simulink model "Final_project"  (R2015b)
settings: Solver=FixedStepDiscrete  StartTime=0.0  StopTime=10.0  RelTol=1e-3
InitFcn:
  | parameters
values from neighbouring files (symbols this model uses):
  Ak = 100    [parameters.m]
  b = 100    [parameters.m]
  dT = 0.01    [parameters.m]
  H = 20    [parameters.m]
  m = 2000    [parameters.m]
  pot_gain = .33    (= 0.33)    [parameters.m]
  pot_offset = 512    [parameters.m]
  R = 1/5    (= 0.2)    [parameters.m]
  V_Ki = 50    [parameters.m]
  V_Kp = 5000    [parameters.m]
undefined symbols (not defined in the file or in its folder): A10, A13, A14, AN0, AN12, B, B13, B4, B6, C6, D, D11, D4, DiscIntNeverNeededParam, F17, F3, F4, G4, H4, L3, PA10, PA11, PA12, PA13, PA14, PA5, PA6, PA7, PA8, PA9, PB10, PB7, PC6, PD10, PD11, PG4, R10, R16, R5, R8, T15
libraries: Conv_Lib x54, rappid_564xl_ec_toolbox x34, Veh_Sim x9, simulink x4, U_of_M_5643_blockset x1
(part 2 of 2)

== system Final_project/High Level Design/Automatic Cruise Control/Speed Ctrl/PI/My Discrete Integrator ==
  X_dot : Inport
  Gain : Gain  Gain=dT  SaturateOnIntegerOverflow=on  OutDataTypeStr=Inherit: Same as input  ParamDataTypeStr=Inherit: Same as input
  Sum : Sum  Inputs=|++  SaturateOnIntegerOverflow=on  InputSameDT=on  OutDataTypeStr=Inherit: Same as first input
  Unit Delay : UnitDelay  SampleTime=-1
  X : Outport
  wires:
  Unit Delay/1 -> X/1, Sum/2
  Sum/1 -> Unit Delay/1
  X_dot/1 -> Gain/1
  Gain/1 -> Sum/1
